simulink model "simulinkCart_"  (R2023b)
settings: Solver=ode4  StartTime=0.0  StopTime=100  FixedStep=0.001  RelTol=1e-3
libraries: simulink x6, slpidlib x2, Controllers x1
settings Model: Creator=calebe  LastModifiedBy=calebe

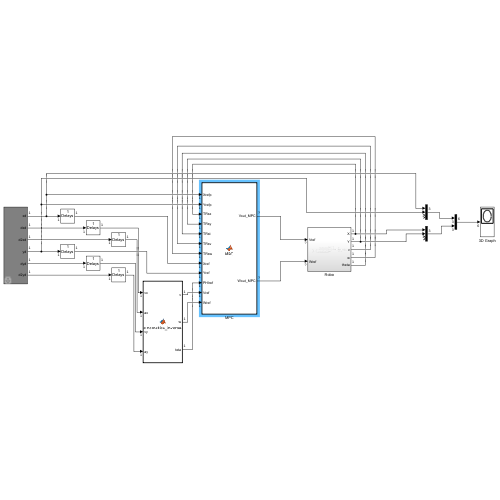
[thumbnail: Simulink's stored preview of the top-level diagram]
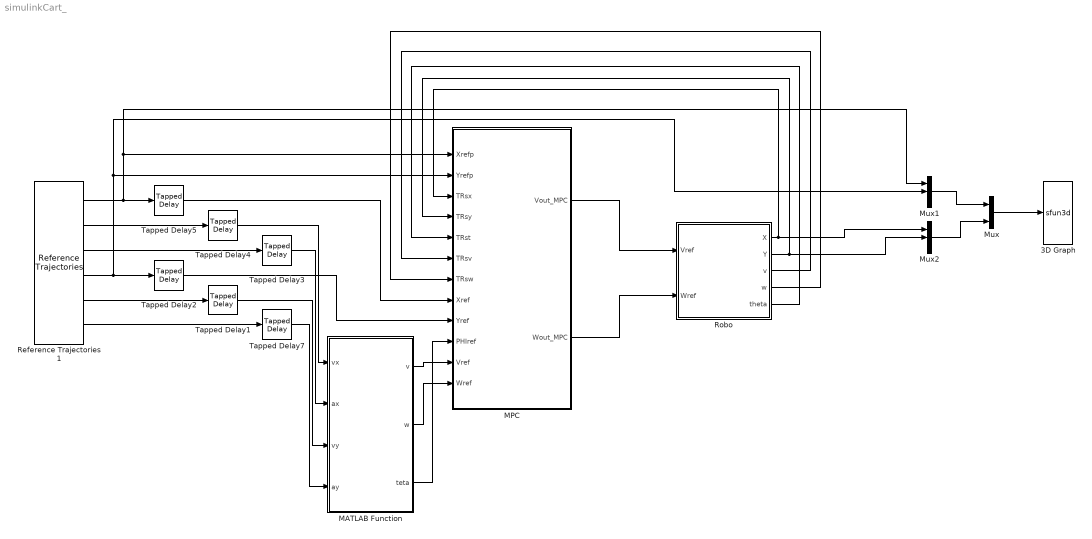
== system simulinkCart_ ==
  3D Graph : S-Function  LoadFcn=if exist('sfun3d','file'), sfun3d([],[],[],'LoadBlock'); end  FunctionName=sfun3d  Parameters=ax,T,np,cp,gd,ls,mk,mx,hd,tb  SFunctionDeploymentMode=off  EnableBusSupport=off  mask(3D Graph){np=2, ax=[-3 3 -3 3 -3 3], mx=1e4, T=0.04, cp=[0 0 1], gd=on, hd=off, tb=off, ls=-, mk=none}
      mask prompts: np "Number of moving points (lines)"; ax "Range: [xmin xmax  ymin ymax zmin zmax]"; mx "Max number of points in each line"; T "Sampling Time"; cp "Camera position (use [0 0 1] for 2D XY view)"; gd "Grid (on|off)"; hd "HeadMarkers (on|off)"; tb "Toolbar (on|off)"; ls "LineStyle"; mk "LineMarker"
      mask help:
      | This block plots the position of several points in the XYZ space. The input contains the coordinates of all the points (x1,y1,z1,x2,y2,z2,...).
      | The number of moving points (lines), the XYZ ranges, sampling time, camera position, and grid (among other things) can be set as mask parameters.
      settings: CopyFcn=if exist('sfun3d','file'), sfun3d([],[],[],'CopyBlock'); end  DeleteFcn=if exist('sfun3d','file'), sfun3d([],[],[],'DeleteBlock'); end  NameChangeFcn=if exist('sfun3d','file'), sfun3d([],[],[],'NameChange'); end
      mask Help:
      | This block plots the position of several points in the XYZ space. The input contains the coordinates of all the points (x1,y1,z1,x2,y2,z2,...).
      | The number of moving points (lines), the XYZ ranges, sampling time, camera position, and grid (among other things) can be set as mask parameters.
      mask TypeOptions ls: - | -- | : | -. | none
      mask TypeOptions mk: none | . | + | o | * | x | square | diamond | v | ^ | > | < | pentagram | hexagram
      mask Display: plot([.05 .95 .95 .05 .05],[.45 .45 .95 .95 .45], 0.5+cos(0:0.1:2*pi)*0.3,0.7+sin(0:0.1:2*pi)*0.2)
  MATLAB Function : MATLAB Function  TreatAsAtomicUnit=on
  MPC : MATLAB Function  TreatAsAtomicUnit=on
  Mux : Mux  Inputs=2
  Mux1 : Mux  Inputs=3
  Mux2 : Mux  Inputs=3
  Reference Trajectories1 : Controllers/Reference Trajectories  trajectory_type=2  wf=0.1  raio_ref_1=1  delta_raio=0  t_delta_raio=60  xd=[1, -1.5]
  Robo : Subsystem
  Tapped Delay{1..5,7} (6 alike) : simulink/Discrete/Tapped Delay  vinit=0.0  samptime=-1  NumDelays=1  DelayOrder=Oldest  includeCurrent=off
  wires:
  MPC/1(Vout_MPC) -> Robo/1(Vref)
  MPC/2(Wout_MPC) -> Robo/2(Wref)
  Mux1/1 -> Mux/1
  Mux2/1 -> Mux/2
  Mux/1 -> 3D Graph/1
  Reference Trajectories1/1 -> MPC/1(Xrefp), Mux1/1, Tapped Delay5/1
  Reference Trajectories1/4 -> MPC/2(Yrefp), Mux1/2, Tapped Delay2/1
  Robo/1(X) -> MPC/3(TRsx), Mux2/1
  Robo/2(Y) -> MPC/4(TRsy), Mux2/2
  Robo/5(theta) -> MPC/5(TRst)
  Robo/3(v) -> MPC/6(TRsv)
  Robo/4(w) -> MPC/7(TRsw)
  Reference Trajectories1/2 -> Tapped Delay4/1
  Reference Trajectories1/3 -> Tapped Delay3/1
  Reference Trajectories1/5 -> Tapped Delay1/1
  Reference Trajectories1/6 -> Tapped Delay7/1
  Tapped Delay5/1 -> MPC/8(Xref)
  Tapped Delay2/1 -> MPC/9(Yref)
  Tapped Delay4/1 -> MATLAB Function/1(vx)
  Tapped Delay3/1 -> MATLAB Function/2(ax)
  Tapped Delay1/1 -> MATLAB Function/3(vy)
  Tapped Delay7/1 -> MATLAB Function/4(ay)
  MATLAB Function/3(teta) -> MPC/10(PHIref)
  MATLAB Function/1(v) -> MPC/11(Vref)
  MATLAB Function/2(w) -> MPC/12(Wref)

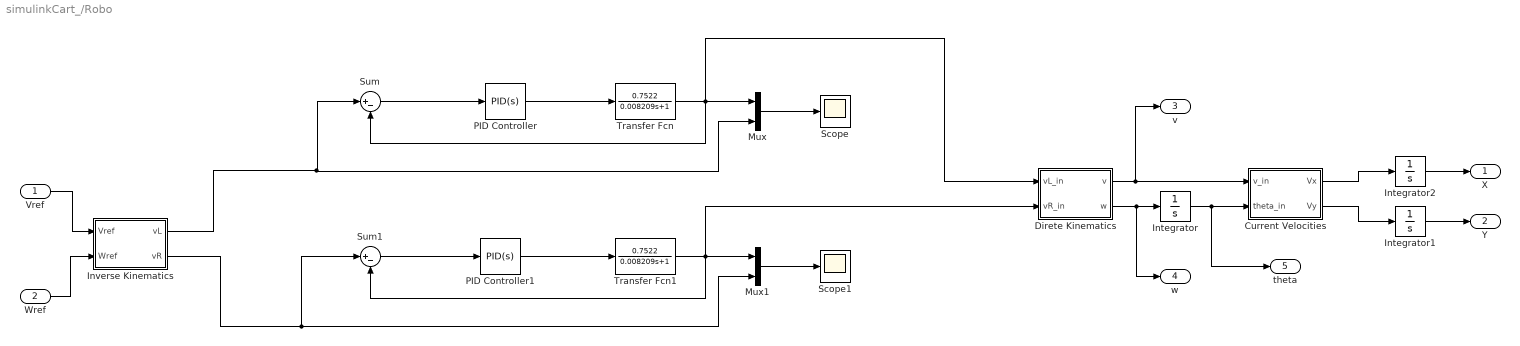
== system simulinkCart_/Robo ==
  Vref : Inport
  Wref : Inport  Port=2
  Current Velocities : MATLAB Function  TreatAsAtomicUnit=on
  Direte Kinematics : MATLAB Function  TreatAsAtomicUnit=on
  Integrator : Integrator
  Integrator1 : Integrator
  Integrator2 : Integrator
  Inverse Kinematics : MATLAB Function  TreatAsAtomicUnit=on
  Mux : Mux  Inputs=2
  Mux1 : Mux  Inputs=2
  PID Controller : slpidlib/PID Controller  Controller=PID  Form=Parallel  TimeDomain=Continuous-time  UseExternalTs=off  SampleTime=-1  IntegratorMethod=Forward Euler  FilterMethod=Forward Euler  ControllerParametersSource=internal  P=20  I=120  UseKiTs=off  D=0  N=460.584925304986  UseFilter=on  TunerSelectOption=Transfer Function Based (PID Tuner App)  InitialConditionSource=internal  InitialConditionForIntegrator=0  InitialConditionForFilter=0  DifferentiatorICPrevScaledInput=0  ExternalReset=none  TrackingMode=off  Kt=1  LimitOutput=off  SatLimitsSource=internal  UpperSaturationLimit=inf  LowerSaturationLimit=-inf  LinearizeAsGain=on  AntiWindupMode=none  Kb=1  LimitIntegrator=off  UpperIntegratorSaturationLimit=inf  LowerIntegratorSaturationLimit=-inf  POutMin=[]  POutMax=[]  IOutMin=[]  IOutMax=[]  DOutMin=[]  DOutMax=[]  NOutMin=[]  NOutMax=[]  SumOutMin=[]  SumOutMax=[]  SaturationOutMin=[]  SaturationOutMax=[]  PParamMin=[]  PParamMax=[]  IParamMin=[]  IParamMax=[]  DParamMin=[]  DParamMax=[]  NParamMin=[]  NParamMax=[]  KbParamMin=[]  KbParamMax=[]  KtParamMin=[]  KtParamMax=[]  KbOutMin=[]  KbOutMax=[]  KtOutMin=[]  KtOutMax=[]  IntegratorOutMin=[]  IntegratorOutMax=[]  FilterOutMin=[]  FilterOutMax=[]  SumI1OutMin=[]  SumI1OutMax=[]  SumI2OutMin=[]  SumI2OutMax=[]  SumI3OutMin=[]  SumI3OutMax=[]  SumI4OutMin=[]  SumI4OutMax=[]  SumDOutMin=[]  SumDOutMax=[]  DifferentiatorOutMin=[]  DifferentiatorOutMax=[]  FilterDiffOutCoefMin=[]  FilterDiffOutCoefMax=[]  ReciprocalOutMin=[]  ReciprocalOutMax=[]  SumDenOutMin=[]  SumDenOutMax=[]  SumNumOutMin=[]  SumNumOutMax=[]  DivideOutMin=[]  DivideOutMax=[]  UdiffTsProdOutMin=[]  UdiffTsProdOutMax=[]  NTsProdOutMin=[]  NTsProdOutMax=[]  UintegralTsProdOutMin=[]  UintegralTsProdOutMax=[]  UngainTsProdOutMin=[]  UngainTsProdOutMax=[]  ClampingZeroOutDataTypeStr=Inherit: Inherit via back propagation  ClampingZeroOutMin=[]  ClampingZeroOutMax=[]  FilterDenConstantOutDataTypeStr=Inherit: Inherit via back propagation  FilterDenConstantOutMin=[]  FilterDenConstantOutMax=[]  PCopyOutDataTypeStr=Inherit: Inherit via back propagation  PCopyOutMin=[]  PCopyOutMax=[]  NCopyOutDataTypeStr=Inherit: Inherit via back propagation  NCopyOutMin=[]  NCopyOutMax=[]  IntegratorContinuousStateAttributes=''  IntegratorStateMustResolveToSignalObject=off  IntegratorRTWStateStorageClass=Auto  FilterContinuousStateAttributes=''  FilterStateMustResolveToSignalObject=off  FilterRTWStateStorageClass=Auto  ParallelPVariant=InternalParameters  IdealPVariant=Disabled  IVariant=InternalParameters  DVariant=InternalParameters  IntegratorVariant=Continuous  SatVariant=Disabled  AWVariant=Passthrough  PCopyVariant=Disabled  TRVariant=Disabled  FdbkBlocksVariant=Forward  IdealPFdbkVariant=Disabled  SatFdbkVariant=Disabled  DerivativeFilterVariant=ContFilter  NVariant=InternalParameters  NCopyVariant=Disabled  FilterICVariant=InternalICsFilter  IntegratorICVariant=InternalICs  ExternalResetVariant=Disabled  TRSumVariant=Passthrough  SumFdbkVariant=Disabled  SumVariant=Sum_PID  TsampFilterVariant=InternalTs  TsampNgainVariant=Passthrough  TsampIntegralVariant=Disabled_SignalSpec  ExternalSaturationOutDataTypeStr=Inherit: Same as second input
  PID Controller1 : slpidlib/PID Controller  Controller=PID  Form=Parallel  TimeDomain=Continuous-time  UseExternalTs=off  SampleTime=-1  IntegratorMethod=Forward Euler  FilterMethod=Forward Euler  ControllerParametersSource=internal  P=20  I=120  UseKiTs=off  D=0  N=460.584925304986  UseFilter=on  TunerSelectOption=Transfer Function Based (PID Tuner App)  InitialConditionSource=internal  InitialConditionForIntegrator=0  InitialConditionForFilter=0  DifferentiatorICPrevScaledInput=0  ExternalReset=none  TrackingMode=off  Kt=1  LimitOutput=off  SatLimitsSource=internal  UpperSaturationLimit=inf  LowerSaturationLimit=-inf  LinearizeAsGain=on  AntiWindupMode=none  Kb=1  LimitIntegrator=off  UpperIntegratorSaturationLimit=inf  LowerIntegratorSaturationLimit=-inf  POutMin=[]  POutMax=[]  IOutMin=[]  IOutMax=[]  DOutMin=[]  DOutMax=[]  NOutMin=[]  NOutMax=[]  SumOutMin=[]  SumOutMax=[]  SaturationOutMin=[]  SaturationOutMax=[]  PParamMin=[]  PParamMax=[]  IParamMin=[]  IParamMax=[]  DParamMin=[]  DParamMax=[]  NParamMin=[]  NParamMax=[]  KbParamMin=[]  KbParamMax=[]  KtParamMin=[]  KtParamMax=[]  KbOutMin=[]  KbOutMax=[]  KtOutMin=[]  KtOutMax=[]  IntegratorOutMin=[]  IntegratorOutMax=[]  FilterOutMin=[]  FilterOutMax=[]  SumI1OutMin=[]  SumI1OutMax=[]  SumI2OutMin=[]  SumI2OutMax=[]  SumI3OutMin=[]  SumI3OutMax=[]  SumI4OutMin=[]  SumI4OutMax=[]  SumDOutMin=[]  SumDOutMax=[]  DifferentiatorOutMin=[]  DifferentiatorOutMax=[]  FilterDiffOutCoefMin=[]  FilterDiffOutCoefMax=[]  ReciprocalOutMin=[]  ReciprocalOutMax=[]  SumDenOutMin=[]  SumDenOutMax=[]  SumNumOutMin=[]  SumNumOutMax=[]  DivideOutMin=[]  DivideOutMax=[]  UdiffTsProdOutMin=[]  UdiffTsProdOutMax=[]  NTsProdOutMin=[]  NTsProdOutMax=[]  UintegralTsProdOutMin=[]  UintegralTsProdOutMax=[]  UngainTsProdOutMin=[]  UngainTsProdOutMax=[]  ClampingZeroOutDataTypeStr=Inherit: Inherit via back propagation  ClampingZeroOutMin=[]  ClampingZeroOutMax=[]  FilterDenConstantOutDataTypeStr=Inherit: Inherit via back propagation  FilterDenConstantOutMin=[]  FilterDenConstantOutMax=[]  PCopyOutDataTypeStr=Inherit: Inherit via back propagation  PCopyOutMin=[]  PCopyOutMax=[]  NCopyOutDataTypeStr=Inherit: Inherit via back propagation  NCopyOutMin=[]  NCopyOutMax=[]  IntegratorContinuousStateAttributes=''  IntegratorStateMustResolveToSignalObject=off  IntegratorRTWStateStorageClass=Auto  FilterContinuousStateAttributes=''  FilterStateMustResolveToSignalObject=off  FilterRTWStateStorageClass=Auto  ParallelPVariant=InternalParameters  IdealPVariant=Disabled  IVariant=InternalParameters  DVariant=InternalParameters  IntegratorVariant=Continuous  SatVariant=Disabled  AWVariant=Passthrough  PCopyVariant=Disabled  TRVariant=Disabled  FdbkBlocksVariant=Forward  IdealPFdbkVariant=Disabled  SatFdbkVariant=Disabled  DerivativeFilterVariant=ContFilter  NVariant=InternalParameters  NCopyVariant=Disabled  FilterICVariant=InternalICsFilter  IntegratorICVariant=InternalICs  ExternalResetVariant=Disabled  TRSumVariant=Passthrough  SumFdbkVariant=Disabled  SumVariant=Sum_PID  TsampFilterVariant=InternalTs  TsampNgainVariant=Passthrough  TsampIntegralVariant=Disabled_SignalSpec  ExternalSaturationOutDataTypeStr=Inherit: Same as second input
  Scope : Scope
  Scope1 : Scope
  Sum : Sum  Inputs=|+-
  Sum1 : Sum  Inputs=|+-
  Transfer Fcn : TransferFcn  Numerator=[0.7522]  Denominator=[0.008209 1]
  Transfer Fcn1 : TransferFcn  Numerator=[0.7522]  Denominator=[0.008209 1]
  X : Outport
  Y : Outport  Port=2
  v : Outport  Port=3
  w : Outport  Port=4
  theta : Outport  Port=5
  wires:
  Sum/1 -> PID Controller/1
  PID Controller/1 -> Transfer Fcn/1
  Mux/1 -> Scope/1
  Inverse Kinematics/1(vL) -> Sum/1, Mux/2
  Mux1/1 -> Scope1/1
  Inverse Kinematics/2(vR) -> Sum1/1, Mux1/2
  Transfer Fcn1/1 -> Direte Kinematics/2(vR_in), Sum1/2, Mux1/1
  PID Controller1/1 -> Transfer Fcn1/1
  Vref/1 -> Inverse Kinematics/1(Vref)
  Wref/1 -> Inverse Kinematics/2(Wref)
  Transfer Fcn/1 -> Direte Kinematics/1(vL_in), Sum/2, Mux/1
  Direte Kinematics/1(v) -> Current Velocities/1(v_in), v/1
  Direte Kinematics/2(w) -> Integrator/1, w/1
  Integrator/1 -> theta/1, Current Velocities/2(theta_in)
  Current Velocities/1(Vx) -> Integrator2/1
  Current Velocities/2(Vy) -> Integrator1/1
  Integrator1/1 -> Y/1
  Integrator2/1 -> X/1
  Sum1/1 -> PID Controller1/1

== matlab function simulinkCart_/Robo/Direte Kinematics ==
  data: vL_in input; v output; vR_in input; w output
function [v, w] = direct(vL_in, vR_in)
%#codegen

% --- Definição dos Parâmetros do Robô ---
% L = Distância entre as rodas (em metros) - PRECISA AJUSTAR DEPOIS!
% Use o MESMO valor que você usou na Inverse Kinematics.
L = 0.115; % Valor temporário, ajuste quando souber o correto

% --- Cinemática Direta (Passo 1) ---
% Calcula a velocidade linear (v) e angular (w) do robô
% a partir da velocidade real das rodas (vL_in, vR_in)

v = (vR_in + vL_in) / 2;
w = (vR_in - vL_in) / L;

end % Fim da função

== matlab function simulinkCart_/Robo/Inverse Kinematics ==
  data: Vref input; vL output; Wref input; vR output
function [vL, vR] = inverse(Vref, Wref)
%#codegen

% --- Definição dos Parâmetros do Robô ---
% L = Distância entre as rodas (em metros) - PRECISA AJUSTAR!
% O Turtlebot padrão usa L=0.23m ou L=0.16m. Verifique o valor correto.
L = 0.115; % Exemplo, ajuste se necessário

% --- Cinemática Inversa ---
% Calcula a velocidade linear necessária para cada roda

vR = Vref + (Wref * L) / 2; % Velocidade da Roda Direita
vL = Vref - (Wref * L) / 2; % Velocidade da Roda Esquerda

end % Fim da função

== matlab function simulinkCart_/Robo/Current Velocities ==
  data: v_in input; Vx output; theta_in input; Vy output
function [Vx, Vy] = velocities(v_in, theta_in)
%#codegen

% --- Cinemática Direta (Passo 2) ---
% Calcula as componentes Vx e Vy da velocidade linear v
% usando o ângulo atual theta do robô.

Vx = v_in * cos(theta_in);
Vy = v_in * sin(theta_in);

end % Fim da função

== matlab function simulinkCart_/MPC ==
  data: Xrefp input; Vout_MPC output; Yrefp input; TRsx input; TRsy input; TRst input; TRsv input; TRsw input; Xref input; Yref input; PHIref input; Vref input; Wref input; Wout_MPC output
function [Vout_MPC,Wout_MPC]=MPC(Xrefp, Yrefp, TRsx, TRsy, TRst,TRsv,TRsw, Xref, Yref, PHIref, Vref, Wref)
%#codegen
% Este é o código completo do "cérebro" MPC, baseado no Passo 20 da Prática 4.
% Esta versão está LIMPA, sem os erros de citação.

% --- Passo 20.a: Configuração dos Parâmetros do Controlador ---
Vmax = 0.4;
d = 0.23;
N1 = 1;
N2 = 10;
Nu = 2;
L1 = 10;
L2 = 2000;
L3 = 0.05;
eta = 0.1;
Imax = 15;
I = 0;
Delta = 0.1;

% --- Passo 20.b: Configuração dos Parâmetros do Otimizador ---
alpha = 0.015;

% --- Passo 20.c: Inicialização dos vetores do Otimizador ---
Jsteps = zeros(8, 1);
Jgrad = zeros(4, 1);
Jgrad_prev = zeros(4, 1);

% --- Passo 20.d: Inicializando modelo do preditor ---
Ubest = zeros(2, 2);
Uref = zeros(2, 2);
Uaux = zeros(2, 2);
SimRob = struct('x', 0, 'y', 0, 'teta', 0, 'v', 0, 'w', 0); 

% --- Passo 20.e: INICIALIZAÇÃO DAS VARIÁVEIS DO CONTROLADOR ---

% 20.e.i: Inicialização da Saída de Controle Desejada
Uref(1,1) = Vref;
Uref(2,1) = Wref;
Uref(1,2) = Vref;
Uref(2,2) = Wref;

% 20.e.ii: Cálculo da Trajetória de Referência
% (Esta função 'calcRefTraj' deve estar no seu .zip)
[tPX,tPY,tPTeta] = calcRefTraj(0.01, TRsx, TRsy, TRst, Xref, Yref, PHIref, Vref, Wref, N2, Xrefp, Yrefp);

% 20.e.iii: Atualiza Modelo do Preditor
SimRob.x = TRsx;
SimRob.y = TRsy;
SimRob.teta = TRst;
SimRob.v = TRsv;
SimRob.w = TRsw;

% --- Passo 20.f: INÍCIO DO LOOP DE CONTROLE ---

% 20.f.i: Satura as Velocidades
% (Esta função 'scaleForSaturation' deve estar no seu .zip)
Uref = scaleForSaturation(Uref, d, Nu, Vmax);

% 20.f.ii: Calcula o Valor Inicial da Função Custo J
Jatual = COST_FUNCTION(SimRob.x, SimRob.y, SimRob.teta, SimRob.v, SimRob.w, Uref, tPX, tPY, tPTeta, N1, N2, Nu, L1, L2, L3);
Jbest = Jatual;
Ubest = Uref;

% 20.f.iii: INÍCIO DO LOOP DE OTIMIZAÇÃO
I = 0; % Zerando o contador I
while (I < Imax && Jatual > eta)
    
    % 20.f.iv: Calcula os Passos (Usteps)
    Usteps = calcUsteps(Uref, Nu, Delta);
    
    % 20.f.v: Cálculo de todos os J para o horizonte
    for k = 0:1:Nu-1
        for j = 1:1:4
            % 1. Atribui velocidades para cada passo
            for m = 0:1:Nu-1
                if m == k
                    Uaux(1,m+1) = Usteps(1,(j+4*k));
                    Uaux(2,m+1) = Usteps(2,(j+4*k));
                else
                    Uaux(1,m+1) = Uref(1,m+1);
                    Uaux(2,m+1) = Uref(2,m+1);
                end
            end
            
            % 2. Reinicia a posição inicial
            SimRob.x = TRsx;
            SimRob.y = TRsy;
            SimRob.teta = TRst;
            SimRob.v = TRsv;
            SimRob.w = TRsw;
            
            % 3. Satura novamente
            % (Esta função 'scaleForSaturation' deve estar no seu .zip)
            Uaux = scaleForSaturation(Uaux, d, Nu, Vmax);
            
            % 4. Calcula o J da iteração
            J = COST_FUNCTION(SimRob.x, SimRob.y, SimRob.teta, SimRob.v, SimRob.w, Uaux, tPX, tPY, tPTeta, N1, N2, Nu, L1, L2, L3);
            Jsteps(j+4*k, 1) = J;
        end
    end
    
    % 20.f.vi: Calcula o Gradiente de J
    for h = 0:1:Nu-1
        Jgrad_prev(2*h+1,1) = Jgrad(2*h+1,1);
        Jgrad(2*h+1,1) = Jsteps(4*h+1,1) - Jsteps(4*h+2,1);
        
        Jgrad_prev(2*h+2,1) = Jgrad(2*h+2,1);
        Jgrad(2*h+2,1) = Jsteps(4*h+3,1) - Jsteps(4*h+4,1);
    end
    
    % 20.f.vii: Cálculo do Gradiente Conjugado
    di = [0 0];
    x1 = di;
    for z = 0:1:Nu-1
        di(1) = Jgrad(2*z+1,1);
        di(2) = Jgrad(2*z+2,1);
        
        x1(1) = (Uref(1,z+1) - alpha*di(1));
        x1(2) = (Uref(2,z+1) - alpha*di(2));
        
        Jgrad_prev(2*z+1,1) = Jgrad(2*z+1,1);
        Jgrad(2*z+1,1) = Jsteps(4*z+1,1) - Jsteps(4*z+2,1);
        Jgrad_prev(2*z+2,1) = Jgrad(2*z+2,1);
        Jgrad(2*z+2,1) = Jsteps(4*z+3,1) - Jsteps(4*z+4,1);
        
        beta = 0;
        if ((Jgrad(2*z+1,1) >= eta) || (Jgrad(2*z+2,1) >= eta))
            t1 = (Jgrad(2*z+1,1) - Jgrad_prev(2*z+1,1));
            t2 = (Jgrad(2*z+2,1) - Jgrad_prev(2*z+2,1));
            a1 = (Jgrad(2*z+1,1) * t1);
            a2 = (Jgrad(2*z+2,1) * t2);
            b1 = (Jgrad_prev(2*z+1,1) * Jgrad_prev(2*z+1,1));
            b2 = (Jgrad_prev(2*z+2,1) * Jgrad_prev(2*z+2,1));
            if (b1+b2) ~= 0 % Evitar divisão por zero
                beta = ((a1+a2)/(b1+b2));
            end
        end
        
        Uref(1,z+1) = x1(1) + alpha*(-Jgrad(2*z+1,1) + beta*Jgrad_prev(2*z+1,1));
        Uref(2,z+1) = x1(2) + alpha*(-Jgrad(2*z+2,1) + beta*Jgrad_prev(2*z+2,1));
    end
    
    % 20.f.viii: Reinicia Posição
    SimRob.x = TRsx;
    SimRob.y = TRsy;
    SimRob.teta = TRst;
    SimRob.v = TRsv;
    SimRob.w = TRsw;
    
    % 20.f.ix: Satura Velocidade
    % (Esta função 'scaleForSaturation' deve estar no seu .zip)
    Uref = scaleForSaturation(Uref, d, Nu, Vmax);
    
    % 20.f.x: Recalcula J Atual
    Jatual = COST_FUNCTION(SimRob.x, SimRob.y, SimRob.teta, SimRob.v, SimRob.w, Uref, tPX, tPY, tPTeta, N1, N2, Nu, L1, L2, L3);
    
    % 20.f.xi: Testa se J é melhor
    if Jatual < Jbest
        Jbest = Jatual;
        Ubest = Uref;
    end
    
    I = I + 1;
end % Fim do loop 'while'

% --- Passo 20.g: SAÍDA DO CONTROLADOR ---
Vout_MPC = Ubest(1, 1);
Wout_MPC = Ubest(2, 1);


% =================================================================
% --- FUNÇÕES LOCAIS (NESTED FUNCTIONS) ---
% =l================================================================

% --- Função COST_FUNCTION (Baseada na descrição 20.f.ii.1-5) ---
function J = COST_FUNCTION(x, y, teta, v, w, U, tPX, tPY, tPTeta, N1, N2, Nu, L1, L2, L3)
    
    % 1. Zera variáveis de soma
    sumX = 0;
    sumY = 0;
    sumT = 0;
    sum_dU = 0;
    
    % Prepara a simulação do robô
    SimRob.x = x;
    SimRob.y = y;
    SimRob.teta = teta;
    
    % 2. Define tempo discreto
    t = 0.01;
    
    % 3. Inicia laço de N1 a N2
    for i = N1:N2
        
        % a. Atribui velocidades
        current_U_index = i;
        if i > Nu
            current_U_index = Nu;
        end
        v_sim = U(1, current_U_index);
        w_sim = U(2, current_U_index);
        
        % b. Inicia laço de simulação interna (4 passos de 0.01s = 0.04s)
        for j = 1:4
            % i. Realiza simulação (slide 44 da aula_3.pdf)
            SimRob.teta = SimRob.teta + w_sim * t;
            SimRob.x = SimRob.x + v_sim * cos(SimRob.teta) * t;
            SimRob.y = SimRob.y + v_sim * sin(SimRob.teta) * t;
        end
        
        % c. Realiza somatório da função custo
        ex = SimRob.x - tPX(i);
        ey = SimRob.y - tPY(i);
        eT = DiffAngle(SimRob.teta, tPTeta(i));
        
        sumX = sumX + ex^2;
        sumY = sumY + ey^2;
        sumT = sumT + eT^2;
    end
    
    % 4. Somatório da variação de velocidades
    for i = 1:Nu-1
        sum_dU = sum_dU + (U(1,i+1) - U(1,i))^2 + (U(2,i+1) - U(2,i))^2;
    end
    
    % 5. Custo Total
    J = L1*(sumX + sumY) + L2*sumT + L3*sum_dU;
end


% --- Função Auxiliar: Diff Angle ---
function[ang] = DiffAngle(a1,a2)
    ang = a1-a2;
    if ang < 0
        ang = -((-ang/(2*pi)) - floor((-ang/(2*pi))) * 2*pi);
    end
    if ang < -pi
        ang = ang + 2*pi;
    else
        ang = ((ang/(2*pi)) - floor((ang/(2*pi)))) * (2*pi);
    end
    if ang > pi
        ang = ang - 2*pi;
    end
end

% --- Função Auxiliar: calcUsteps ---
function[dU] = calcUsteps(U, Nu, delta)
    dU = zeros(2,(Nu*4));
    for i=0:1:Nu-1
        dU(1,1+4*i) = U(1,i+1) + delta;
        dU(2,1+4*i) = U(2,i+1);
        
        dU(1,2+4*i) = U(1,i+1) - delta;
        dU(2,2+4*i) = U(2,i+1);
        
        dU(1,3+4*i) = U(1,i+1);
        dU(2,3+4*i) = U(2,i+1) + delta;
        
        dU(1,4+4*i) = U(1,i+1);
        dU(2,4+4*i) = U(2,i+1) - delta;
    end
end


end % <--- ESTE É O 'END' FINAL QUE FECHA A FUNÇÃO 'MPC'

== matlab function simulinkCart_/MATLAB Function ==
  data: vx input; v output; ax input; vy input; ay input; w output; teta output
function [v, w, teta] = cinematica_inversa(vx, ax, vy, ay)
%#codegen
% Este bloco implementa a Cinemática Inversa do Passo 17
% Entradas: [vx, ax, vy, ay] (velocidades e acelerações do Mundo)
% Saídas: [v, w, teta] (velocidades e ângulo do Robô)

% Fórmula para 'v' (Velocidade Linear)
% v = sqrt(vx^2 + vy^2)
% (aula_3.pdf, slide 44-45)
v = sqrt(vx^2 + vy^2);

% Fórmula para 'teta' (Ângulo do Robô)
% teta = atan2(vy, vx)
% (aula_3.pdf, slide 44-45)
teta = atan2(vy, vx);

% Fórmula para 'w' (Velocidade Angular)
% w = (ay*vx - ax*vy) / (vx^2 + vy^2)
% (aula_3.pdf, slide 44-45)
if (v < 0.001)
    % Evita divisão por zero se a velocidade for muito baixa
    w = 0;
else
    w = (ay*vx - ax*vy) / (vx^2 + vy^2);
end

end
